simulink library "intraSpoolNetZeroPI_cl"  (R2018b)
settings: Solver=VariableStepAuto  StartTime=0.0  StopTime=10.0  RelTol=1e-3
undefined symbols (not defined in the file or in its folder): pathCtrl
libraries: firstOrderFilter_ul x1, runningAvg_ul x1
settings Model: Creator=James Reed  LastModifiedBy=mcobb

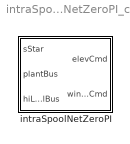
== system intraSpoolNetZeroPI_cl ==
  intraSpoolNetZeroPI : Subsystem

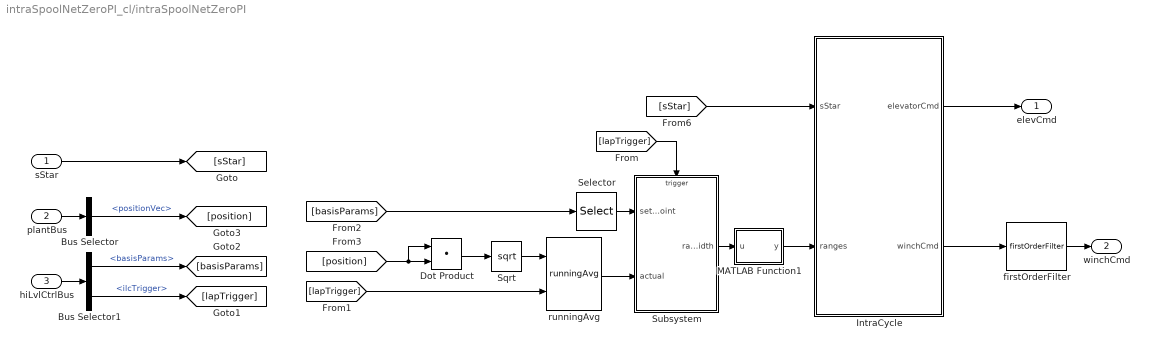
== system intraSpoolNetZeroPI_cl/intraSpoolNetZeroPI ==
  "sStar " : Inport
  plantBus : Inport  Port=2  OutDataTypeStr=Bus: plantBus
  hiLvlCtrlBus : Inport  Port=3  OutDataTypeStr=Bus: hiLvlCtrlBus
  Bus Selector : BusSelector  OutputSignals=positionVec
  Bus Selector1 : BusSelector  OutputSignals=basisParams,ilcTrigger
  Dot Product : DotProduct  InputSameDT=on  OutDataTypeStr=Inherit: Inherit via internal rule
  IntraCycle : Stateflow chart  TreatAsAtomicUnit=on  mask{reelInSpd=pathCtrl.winchSpeedIn.Value, reelOutSpd=pathCtrl.winchSpeedOut.Value, elevatorReelInDef=pathCtrl.elevatorReelInDef.Value}
      mask prompts: reelInSpd "Spool in speed"; reelOutSpd "Spool out speed"; elevatorReelInDef "Elevator Defection during Spool In"
  MATLAB Function1 : MATLAB Function  TreatAsAtomicUnit=on
  Selector : Selector  InputPortWidth=5  IndexOptions=Index vector (dialog)  Indices=5  OutputSizes=1
  Sqrt : Sqrt  SaturateOnIntegerOverflow=on
  Subsystem : Subsystem  mask{ki=0, kp=0}
      mask TypeOptions ki: ki/Gain
      mask TypeOptions kp: kp/Gain
  firstOrderFilter : firstOrderFilter_ul/firstOrderFilter  tau=1  ic=0
  runningAvg : runningAvg_ul/runningAvg  SystemSampleTime=-1
  elevCmd : Outport
  "winchCmd " : Outport  Port=2
  wires:
  firstOrderFilter/1 -> "winchCmd "/1
  [sStar] -> IntraCycle/1(sStar)
  IntraCycle/1(elevatorCmd) -> elevCmd/1
  IntraCycle/2(winchCmd) -> firstOrderFilter/1
  "sStar "/1 -> [sStar]
  Subsystem/1(rangeHalfWidth) -> MATLAB Function1/1(u)
  MATLAB Function1/1(y) -> IntraCycle/2(ranges)
  hiLvlCtrlBus/1 -> Bus Selector1/1
  Selector/1 -> Subsystem/1(setpoint)
  Dot Product/1 -> Sqrt/1
  [position] -> Dot Product/1, Dot Product/2
  Sqrt/1 -> runningAvg/1
  runningAvg/1 -> Subsystem/2(actual)
  [lapTrigger] -> Subsystem/Trigger
  [lapTrigger] -> runningAvg/2
  [basisParams] -> Selector/1
  plantBus/1 -> Bus Selector/1
  Bus Selector/1 -> [position]  "<positionVec>"
  Bus Selector1/1 -> [basisParams]  "<basisParams>"
  Bus Selector1/2 -> [lapTrigger]  "<ilcTrigger>"

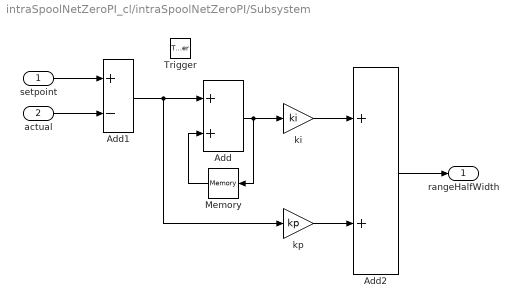
== system intraSpoolNetZeroPI_cl/intraSpoolNetZeroPI/Subsystem ==
  setpoint : Inport
  actual : Inport  Port=2
  Trigger : TriggerPort  VariantControl=Variant  PortDimensions=1
  Add : Sum
  Add1 : Sum  Inputs=+-
  Add2 : Sum
  Memory : Memory
  ki : Gain  Gain=ki
  kp : Gain  Gain=kp
  rangeHalfWidth : Outport
  wires:
  setpoint/1 -> Add1/1
  Memory/1 -> Add/2
  Add/1 -> ki/1, Memory/1
  ki/1 -> Add2/1
  actual/1 -> Add1/2
  kp/1 -> Add2/2
  Add1/1 -> kp/1, Add/1
  Add2/1 -> rangeHalfWidth/1

== stateflow chart intraSpoolNetZeroPI_cl/intraSpoolNetZeroPI/IntraCycle ==
  state ReelOut
    entry:
    winchCmd = reelOutSpd;
    elevatorCmd= 0;
  state ReelIn
    entry:
    elevatorCmd= elevatorReelInDef;
    winchCmd = reelInSpd;
  (default) -> ReelOut
  ReelIn -> ReelOut : [any(and(sStar>=ranges(:,1),sStar<ranges(:,2)))]
  ReelOut -> ReelIn : [ ~any(and(sStar>=ranges(:,1),sStar<ranges(:,2)))]
  data: elevatorCmd output; sStar input; winchCmd output; elevatorReelInDef parameter; reelInSpd parameter; reelOutSpd parameter; ranges input

== matlab function intraSpoolNetZeroPI_cl/intraSpoolNetZeroPI/MATLAB Function1 ==
  data: u input; y output
function y = fcn(u)

y = [...
    0       0.25-u;...
    0.25+u  0.75-u;...
    0.75+u  1];
